simulink model "PedalMappingNoRegen_BPPS"  (R2020a)
settings: Solver=FixedStepDiscrete  StartTime=0.0  StopTime=Inf  FixedStep=Ts  RelTol=1e-3
PostLoadFcn:
  | , if any(exist('dsrtsu_mdlpostloadfcn', 'file') == [2, 3, 6]), try dsrtsu_mdlpostloadfcn('Execute', bdroot); catch fprintf('Error in PostLoadFcn (dsrtsu_mdlpostloadfcn) for model "%s":\n %s\n', bdroot, lasterr); end, end,
InitFcn:
  | , if any(exist('rtifpga_mdlclblib', 'file') ~= 0), rtifpga_mdlclblib('Init', bdroot); end,
Description:
  | Standard RTI1401 template.
  | Supported MATLAB version:  R2018b.
settings Model: Tag=RTI1401  DSRTSU_INTERNAL_RTI_VER=560  DSRTSU_INTERNAL_RTI_TYPE=rti1401  RTICANMMDATA=struct('GeneralSetupData',struct('modelroot','C:\Users\harjo\Git\MACFormulaGit\MicroAutobox\rings\Vehicle_Dynamics_Ring','generalsettings',struct('filesettings',struct('destfolder',struct('Name','RTICANMM_FILES','Check',1),'buildfolder',struct('Name','.','Check',1),'AbsDestfolder',struct('Name','C:\Users\harjo\Git\MACFormulaGit\MicroAutobox\rings\Vehicle_Dynamics_Ring\RTICANMM_FILES'),'AbsBuildfolder',struct('Name','C:\Users\harjo\Git\MACFormulaGit\MicroAutobox\rings\Vehicle_Dynamics_Ring'))),'options',struct('addpaths',1,'rmpaths',1,'addtrcexclusion',true,'cannavigator',struct('checkmonitoring',0),'show_usrtrc',0,'use_usrtrc',0),'advanced',struct('options',ones(1,100)),'MPSetup',{{}},'RTI',struct('Type','RTI1401','Ver','7.14','Date','02-May-2020'),'modelname','PedalMappingNoRegen_BPPS','block','PedalMappingNoRegen_BPPS'))  DSRTSU_INTERNAL_RTIFPGA=160  Creator=Harjot  LastModifiedBy=Harjot
settings OptimizationCC: BlockReduction=off  OptimizeBlockIOStorage=off  BufferReuse=off  GlobalBufferReuse=off  ExpressionFolding=off  LocalBlockOutputs=off  OptimizeDataStoreBuffers=off  BusAssignmentInplaceUpdate=off
settings DebuggingCC: ArithmeticOperatorsInVariantConditions=warning
settings HardwareCC: ProdBitPerPointer=32  ProdBitPerSizeT=32  ProdBitPerPtrDiffT=32  ProdLargestAtomicInteger=Integer  ProdEndianess=BigEndian  ProdWordSize=32  ProdHWDeviceType=Custom Processor->Custom  TargetIntDivRoundTo=Zero  TargetEndianess=BigEndian  TargetHWDeviceType=Custom Processor->Custom
settings SFSimCC: SimUseLocalCustomCode=off  MATLABDynamicMemAlloc=off  CustomCodeUndefinedFunction=UseInterfaceOnly
settings RTWCC: Description=dSPACE DS1401 Hardware Platform  SystemTargetFile=rti1401.tlc  MakeCommand=make_rti  TemplateMakefile=rti1401.tmf  RTWUseLocalCustomCode=off
settings CodeAppCC: StateflowObjectComments=on
settings STFCustomTargetCC: ParMdlRefBuildCompliant=on  MatFileLogging=on  SystemTargetFile=rti1401.tlc
settings GRTTargetCC: TargetLangStandard=C89/C90 (ANSI)  CompOptLevelCompliant=off  ConcurrentExecutionCompliant=off  CombineOutputUpdateFcns=off  CPPClassGenCompliant=off  UseToolchainInfoCompliant=off
settings ConfigComp: CovMetricSettings=dswe

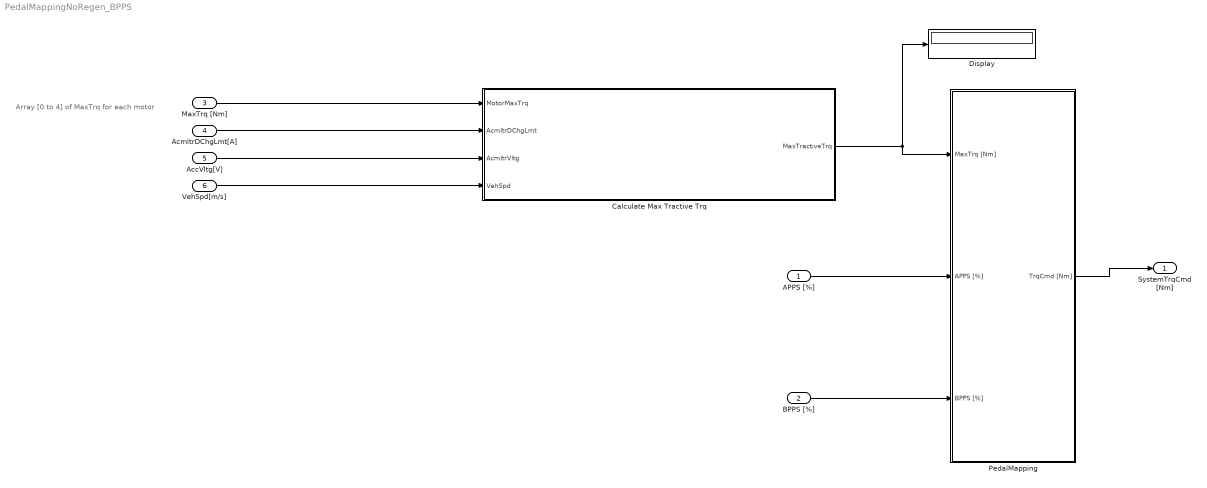
== system PedalMappingNoRegen_BPPS ==
  note: Array [0 to 4] of MaxTrq for each motor
  APPS [%] : Inport
  BPPS [%] : Inport  Port=2
  MaxTrq [Nm] : Inport  Port=3
  AcmltrDChgLmt[A] : Inport  Port=4
  AccVltg[V] : Inport  Port=5
  VehSpd[m/s] : Inport  Port=6
  Calculate Max Tractive Trq : Subsystem
  Display : Display
  PedalMapping : Subsystem
  SystemTrqCmd [Nm] : Outport  VectorParamsAs1DForOutWhenUnconnected=off
  wires:
  MaxTrq [Nm]/1 -> Calculate Max Tractive Trq/1(MotorMaxTrq)
  PedalMapping/1(TrqCmd [Nm]) -> SystemTrqCmd [Nm]/1
  Calculate Max Tractive Trq/1(MaxTractiveTrq) -> PedalMapping/1(MaxTrq [Nm]), Display/1
  AcmltrDChgLmt[A]/1 -> Calculate Max Tractive Trq/2(AcmltrDChgLmt)
  BPPS [%]/1 -> PedalMapping/3(BPPS [%])
  VehSpd[m/s]/1 -> Calculate Max Tractive Trq/4(VehSpd)
  APPS [%]/1 -> PedalMapping/2(APPS [%])
  AccVltg[V]/1 -> Calculate Max Tractive Trq/3(AcmltrVltg)

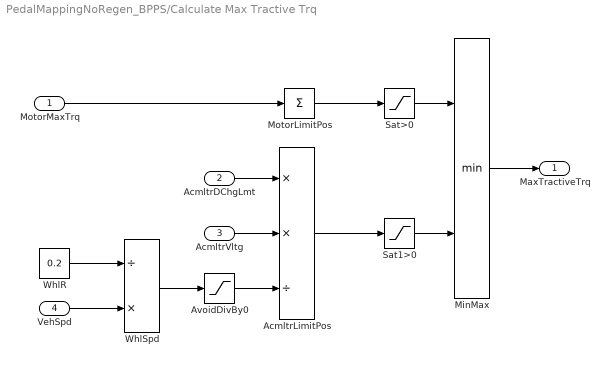
== system PedalMappingNoRegen_BPPS/Calculate Max Tractive Trq ==
  MotorMaxTrq : Inport
  AcmltrDChgLmt : Inport  Port=2
  AcmltrVltg : Inport  Port=3
  VehSpd : Inport  Port=4
  AcmltrLimitPos : Product  Inputs=**/  OutDataTypeStr=double
  AvoidDivBy0 : Saturate  UpperLimit=inf  LowerLimit=1E-7
  MinMax : MinMax  Inputs=2
  MotorLimitPos : Sum  Inputs=+
  Sat1>0 : Saturate  UpperLimit=100000  LowerLimit=0
  Sat>0 : Saturate  UpperLimit=inf  LowerLimit=0
  WhlR : Constant  Value=0.2
  WhlSpd : Product  Inputs=/*
  MaxTractiveTrq : Outport  VectorParamsAs1DForOutWhenUnconnected=off
  wires:
  AcmltrLimitPos/1 -> Sat1>0/1
  AvoidDivBy0/1 -> AcmltrLimitPos/3
  WhlR/1 -> WhlSpd/1
  WhlSpd/1 -> AvoidDivBy0/1
  VehSpd/1 -> WhlSpd/2
  Sat1>0/1 -> MinMax/2
  Sat>0/1 -> MinMax/1
  MotorLimitPos/1 -> Sat>0/1
  AcmltrVltg/1 -> AcmltrLimitPos/2
  AcmltrDChgLmt/1 -> AcmltrLimitPos/1
  MotorMaxTrq/1 -> MotorLimitPos/1
  MinMax/1 -> MaxTractiveTrq/1

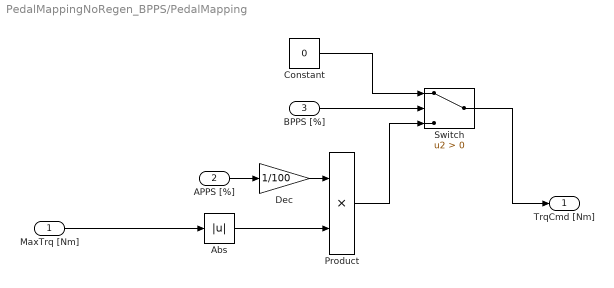
== system PedalMappingNoRegen_BPPS/PedalMapping ==
  MaxTrq [Nm] : Inport
  APPS [%] : Inport  Port=2
  BPPS [%] : Inport  Port=3
  Abs : Abs
  Constant : Constant  Value=0
  Dec : Gain  Gain=1/100
  Product : Product
  Switch : Switch  Criteria=u2 > Threshold
  TrqCmd [Nm] : Outport  VectorParamsAs1DForOutWhenUnconnected=off
  wires:
  Dec/1 -> Product/1
  Abs/1 -> Product/2
  Product/1 -> Switch/3
  APPS [%]/1 -> Dec/1
  MaxTrq [Nm]/1 -> Abs/1
  BPPS [%]/1 -> Switch/2
  Constant/1 -> Switch/1
  Switch/1 -> TrqCmd [Nm]/1
